simulink model "nonlineardtm"  (R2018b)
settings: configuration reference "Physics" (kept outside this file)
model workspace (MAT data in the model file):
  MCOS : class17 (value not decoded)
undefined symbols (not defined in the file): Aerodynamics, Aligning, Antisway, Brakes, Compliance, ContactPatch, Environment, k1_TireFB_PT1, k1_WheelsFB_PT1, k2_TireFB_PT1, Kinematics, Lateral, Longitudinal, normalizeAngle, omega0_K_Vehicle_radps, omega0_Wheels_radps, Overturning, p_Tires_Pa, Rolling, Scaling, SensorData, Structural, TireSimulation, Turnslip, v0_K_Vehicle_mps, v0z_Wheels_mps, VehicleData, Vertical, Wheels, x0_verticaldynamics, z0_TireDeflection_m
libraries: vehdynlibtire x4, vehdynlibsuspension x2, vrlib x1, vehdynlibeom x1
(part 5 of 5)

== system nonlineardtm/Nonlinear Dual Track Model/Subsystem11/Subsystem10 ==
  Alpha : Inport
  Reshape2 : Reshape  OutputDimensionality=Row vector (2-D)
  Selector : Selector  NumberOfDimensions=2  InputPortWidth=12  IndexOptions=Index vector (dialog),Index vector (dialog)  Indices=[1],1  OutputSizes=1,1
  Selector1 : Selector  NumberOfDimensions=2  InputPortWidth=12  IndexOptions=Index vector (dialog),Index vector (dialog)  Indices=1,2  OutputSizes=1,1
  Selector2 : Selector  NumberOfDimensions=2  InputPortWidth=12  IndexOptions=Index vector (dialog),Index vector (dialog)  Indices=1,3  OutputSizes=1,1
  Selector3 : Selector  NumberOfDimensions=2  InputPortWidth=12  IndexOptions=Index vector (dialog),Index vector (dialog)  Indices=1,3  OutputSizes=1,1
  Transfer Fcn1 : TransferFcn  Denominator=[k1_TireFB_PT1(2) 1]
  Transfer Fcn10 : TransferFcn  Denominator=[k1_TireFB_PT1(1) 1]
  Transfer Fcn11 : TransferFcn  Denominator=[k1_TireFB_PT1(1) 1]
  Transfer Fcn9 : TransferFcn  Denominator=[k1_TireFB_PT1(2) 1]
  Vector Concatenate : Concatenate  NumInputs=4
  alpha_ji_rad : Outport
  wires:
  Transfer Fcn1/1 -> Vector Concatenate/4
  Selector3/1 -> Transfer Fcn1/1
  Transfer Fcn9/1 -> Vector Concatenate/3
  Reshape2/1 -> alpha_ji_rad/1
  Alpha/1 -> Selector/1, Selector1/1, Selector2/1, Selector3/1
  Selector/1 -> Transfer Fcn11/1
  Selector2/1 -> Transfer Fcn9/1
  Selector1/1 -> Transfer Fcn10/1
  Transfer Fcn11/1 -> Vector Concatenate/1
  Transfer Fcn10/1 -> Vector Concatenate/2
  Vector Concatenate/1 -> Reshape2/1

== system nonlineardtm/Nonlinear Dual Track Model/Subsystem11/Subsystem14 ==
  z : Inport
  Reshape2 : Reshape  OutputDimensionality=Row vector (2-D)
  Selector : Selector  NumberOfDimensions=2  InputPortWidth=12  IndexOptions=Index vector (dialog),Index vector (dialog)  Indices=[1],1  OutputSizes=1,1
  Selector1 : Selector  NumberOfDimensions=2  InputPortWidth=12  IndexOptions=Index vector (dialog),Index vector (dialog)  Indices=1,2  OutputSizes=1,1
  Selector2 : Selector  NumberOfDimensions=2  InputPortWidth=12  IndexOptions=Index vector (dialog),Index vector (dialog)  Indices=1,3  OutputSizes=1,1
  Selector3 : Selector  NumberOfDimensions=2  InputPortWidth=12  IndexOptions=Index vector (dialog),Index vector (dialog)  Indices=1,3  OutputSizes=1,1
  Transfer Fcn1 : TransferFcn  Denominator=[k2_TireFB_PT1(2) 1]
  Transfer Fcn10 : TransferFcn  Denominator=[k2_TireFB_PT1(1) 1]
  Transfer Fcn11 : TransferFcn  Denominator=[k2_TireFB_PT1(1) 1]
  Transfer Fcn9 : TransferFcn  Denominator=[k2_TireFB_PT1(2) 1]
  Vector Concatenate : Concatenate  NumInputs=4
  rz_Tji_Rji_m : Outport
  wires:
  Vector Concatenate/1 -> Reshape2/1
  Transfer Fcn10/1 -> Vector Concatenate/2
  Transfer Fcn11/1 -> Vector Concatenate/1
  Selector1/1 -> Transfer Fcn10/1
  Selector2/1 -> Transfer Fcn9/1
  Selector/1 -> Transfer Fcn11/1
  z/1 -> Selector3/1, Selector2/1, Selector1/1, Selector/1
  Reshape2/1 -> rz_Tji_Rji_m/1
  Transfer Fcn9/1 -> Vector Concatenate/3
  Selector3/1 -> Transfer Fcn1/1
  Transfer Fcn1/1 -> Vector Concatenate/4

== system nonlineardtm/Nonlinear Dual Track Model/Subsystem11/Subsystem2 ==
  zdot : Inport
  Reshape2 : Reshape  OutputDimensionality=Row vector (2-D)
  Selector : Selector  NumberOfDimensions=2  InputPortWidth=12  IndexOptions=Index vector (dialog),Index vector (dialog)  Indices=[1],1  OutputSizes=1,1
  Selector1 : Selector  NumberOfDimensions=2  InputPortWidth=12  IndexOptions=Index vector (dialog),Index vector (dialog)  Indices=1,2  OutputSizes=1,1
  Selector2 : Selector  NumberOfDimensions=2  InputPortWidth=12  IndexOptions=Index vector (dialog),Index vector (dialog)  Indices=1,3  OutputSizes=1,1
  Selector3 : Selector  NumberOfDimensions=2  InputPortWidth=12  IndexOptions=Index vector (dialog),Index vector (dialog)  Indices=1,3  OutputSizes=1,1
  Transfer Fcn1 : TransferFcn  Denominator=[k2_TireFB_PT1(2) 1]
  Transfer Fcn10 : TransferFcn  Denominator=[k2_TireFB_PT1(1) 1]
  Transfer Fcn11 : TransferFcn  Denominator=[k2_TireFB_PT1(1) 1]
  Transfer Fcn9 : TransferFcn  Denominator=[k2_TireFB_PT1(2) 1]
  Vector Concatenate : Concatenate  NumInputs=4
  vz_Tji_Rji_mps : Outport
  wires:
  Transfer Fcn1/1 -> Vector Concatenate/4
  Selector3/1 -> Transfer Fcn1/1
  Transfer Fcn9/1 -> Vector Concatenate/3
  Reshape2/1 -> vz_Tji_Rji_mps/1
  zdot/1 -> Selector/1, Selector1/1, Selector2/1, Selector3/1
  Selector/1 -> Transfer Fcn11/1
  Selector2/1 -> Transfer Fcn9/1
  Selector1/1 -> Transfer Fcn10/1
  Transfer Fcn11/1 -> Vector Concatenate/1
  Transfer Fcn10/1 -> Vector Concatenate/2
  Vector Concatenate/1 -> Reshape2/1

== system nonlineardtm/Nonlinear Dual Track Model/Subsystem11/Subsystem3 ==
  Re : Inport
  Reshape2 : Reshape  OutputDimensionality=Row vector (2-D)
  Selector : Selector  NumberOfDimensions=2  InputPortWidth=12  IndexOptions=Index vector (dialog),Index vector (dialog)  Indices=[1],1  OutputSizes=1,1
  Selector1 : Selector  NumberOfDimensions=2  InputPortWidth=12  IndexOptions=Index vector (dialog),Index vector (dialog)  Indices=1,2  OutputSizes=1,1
  Selector2 : Selector  NumberOfDimensions=2  InputPortWidth=12  IndexOptions=Index vector (dialog),Index vector (dialog)  Indices=1,3  OutputSizes=1,1
  Selector3 : Selector  NumberOfDimensions=2  InputPortWidth=12  IndexOptions=Index vector (dialog),Index vector (dialog)  Indices=1,3  OutputSizes=1,1
  Transfer Fcn1 : TransferFcn  Denominator=[k2_TireFB_PT1(2) 1]
  Transfer Fcn10 : TransferFcn  Denominator=[k2_TireFB_PT1(1) 1]
  Transfer Fcn11 : TransferFcn  Denominator=[k2_TireFB_PT1(1) 1]
  Transfer Fcn9 : TransferFcn  Denominator=[k2_TireFB_PT1(2) 1]
  Vector Concatenate : Concatenate  NumInputs=4
  re_ji_m : Outport
  wires:
  Vector Concatenate/1 -> Reshape2/1
  Transfer Fcn10/1 -> Vector Concatenate/2
  Transfer Fcn11/1 -> Vector Concatenate/1
  Selector1/1 -> Transfer Fcn10/1
  Selector2/1 -> Transfer Fcn9/1
  Selector/1 -> Transfer Fcn11/1
  Re/1 -> Selector3/1, Selector2/1, Selector1/1, Selector/1
  Reshape2/1 -> re_ji_m/1
  Transfer Fcn9/1 -> Vector Concatenate/3
  Selector3/1 -> Transfer Fcn1/1
  Transfer Fcn1/1 -> Vector Concatenate/4

== system nonlineardtm/Nonlinear Dual Track Model/Subsystem11/Subsystem6 ==
  F : Inport
  Matrix Concatenate : Concatenate  NumInputs=3  Mode=Multidimensional array
  Reshape2 : Reshape  OutputDimensionality=Row vector (2-D)
  Reshape3 : Reshape  OutputDimensionality=Row vector (2-D)
  Reshape4 : Reshape  OutputDimensionality=Row vector (2-D)
  Selector : Selector  NumberOfDimensions=2  InputPortWidth=12  IndexOptions=Index vector (dialog),Index vector (dialog)  Indices=[1],1  OutputSizes=1,1
  Selector1 : Selector  NumberOfDimensions=2  InputPortWidth=12  IndexOptions=Index vector (dialog),Index vector (dialog)  Indices=1,2  OutputSizes=1,1
  Selector12 : Selector  NumberOfDimensions=2  InputPortWidth=12  IndexOptions=Index vector (dialog),Index vector (dialog)  Indices=2,1  OutputSizes=1,1
  Selector13 : Selector  NumberOfDimensions=2  InputPortWidth=12  IndexOptions=Index vector (dialog),Index vector (dialog)  Indices=2,2  OutputSizes=1,1
  Selector14 : Selector  NumberOfDimensions=2  InputPortWidth=12  IndexOptions=Index vector (dialog),Index vector (dialog)  Indices=2,3  OutputSizes=1,1
  Selector15 : Selector  NumberOfDimensions=2  InputPortWidth=12  IndexOptions=Index vector (dialog),Index vector (dialog)  Indices=2,4  OutputSizes=1,1
  Selector16 : Selector  NumberOfDimensions=2  InputPortWidth=12  IndexOptions=Index vector (dialog),Index vector (dialog)  Indices=3,1  OutputSizes=1,1
  Selector17 : Selector  NumberOfDimensions=2  InputPortWidth=12  IndexOptions=Index vector (dialog),Index vector (dialog)  Indices=3,2  OutputSizes=1,1
  Selector18 : Selector  NumberOfDimensions=2  InputPortWidth=12  IndexOptions=Index vector (dialog),Index vector (dialog)  Indices=3,3  OutputSizes=1,1
  Selector19 : Selector  NumberOfDimensions=2  InputPortWidth=12  IndexOptions=Index vector (dialog),Index vector (dialog)  Indices=3,4  OutputSizes=1,1
  Selector2 : Selector  NumberOfDimensions=2  InputPortWidth=12  IndexOptions=Index vector (dialog),Index vector (dialog)  Indices=1,3  OutputSizes=1,1
  Selector3 : Selector  NumberOfDimensions=2  InputPortWidth=12  IndexOptions=Index vector (dialog),Index vector (dialog)  Indices=1,4  OutputSizes=1,1
  Transfer Fcn{1,4..5,8..9,11} (6 alike) : TransferFcn  Denominator=[k1_TireFB_PT1(1) 1]
  Transfer Fcn{2..3,6..7,10,12} (6 alike) : TransferFcn  Denominator=[k1_TireFB_PT1(2) 1]
  Vector Concatenate : Concatenate  NumInputs=4
  Vector Concatenate1 : Concatenate  NumInputs=4
  Vector Concatenate2 : Concatenate  NumInputs=4
  F_Tji_Tji_N : Outport
  wires:
  Reshape4/1 -> Matrix Concatenate/3
  Reshape3/1 -> Matrix Concatenate/2
  Reshape2/1 -> Matrix Concatenate/1
  Vector Concatenate2/1 -> Reshape4/1
  Vector Concatenate1/1 -> Reshape3/1
  Vector Concatenate/1 -> Reshape2/1
  Transfer Fcn6/1 -> Vector Concatenate1/3
  Transfer Fcn7/1 -> Vector Concatenate1/4
  Transfer Fcn8/1 -> Vector Concatenate2/1
  Transfer Fcn9/1 -> Vector Concatenate2/2
  Transfer Fcn12/1 -> Vector Concatenate2/4
  Transfer Fcn10/1 -> Vector Concatenate2/3
  Transfer Fcn5/1 -> Vector Concatenate1/2
  Transfer Fcn4/1 -> Vector Concatenate1/1
  Transfer Fcn3/1 -> Vector Concatenate/4
  Transfer Fcn2/1 -> Vector Concatenate/3
  Transfer Fcn1/1 -> Vector Concatenate/2
  Transfer Fcn11/1 -> Vector Concatenate/1
  Selector19/1 -> Transfer Fcn12/1
  Selector18/1 -> Transfer Fcn10/1
  Selector17/1 -> Transfer Fcn9/1
  Selector16/1 -> Transfer Fcn8/1
  Selector12/1 -> Transfer Fcn4/1
  Selector13/1 -> Transfer Fcn5/1
  Selector14/1 -> Transfer Fcn6/1
  Selector15/1 -> Transfer Fcn7/1
  Selector3/1 -> Transfer Fcn3/1
  Selector1/1 -> Transfer Fcn1/1
  Selector2/1 -> Transfer Fcn2/1
  Selector/1 -> Transfer Fcn11/1
  F/1 -> Selector1/1, Selector2/1, Selector3/1, Selector19/1, Selector18/1, Selector17/1, Selector16/1, Selector15/1, Selector14/1, Selector13/1, Selector12/1, Selector/1
  Matrix Concatenate/1 -> F_Tji_Tji_N/1

== system nonlineardtm/Nonlinear Dual Track Model/Subsystem11/Subsystem8 ==
  omega : Inport
  Reshape2 : Reshape  OutputDimensionality=Row vector (2-D)
  Selector : Selector  NumberOfDimensions=2  InputPortWidth=12  IndexOptions=Index vector (dialog),Index vector (dialog)  Indices=[1],1  OutputSizes=1,1
  Selector1 : Selector  NumberOfDimensions=2  InputPortWidth=12  IndexOptions=Index vector (dialog),Index vector (dialog)  Indices=1,2  OutputSizes=1,1
  Selector2 : Selector  NumberOfDimensions=2  InputPortWidth=12  IndexOptions=Index vector (dialog),Index vector (dialog)  Indices=1,3  OutputSizes=1,1
  Selector3 : Selector  NumberOfDimensions=2  InputPortWidth=12  IndexOptions=Index vector (dialog),Index vector (dialog)  Indices=1,4  OutputSizes=1,1
  Transfer Fcn1 : TransferFcn  Denominator=[k1_WheelsFB_PT1(2) 1]
  Transfer Fcn10 : TransferFcn  Denominator=[k1_WheelsFB_PT1(1) 1]
  Transfer Fcn11 : TransferFcn  Denominator=[k1_WheelsFB_PT1(1) 1]
  Transfer Fcn9 : TransferFcn  Denominator=[k1_WheelsFB_PT1(2) 1]
  Vector Concatenate : Concatenate  NumInputs=4
  omegay_Rji_Rji_radps : Outport
  wires:
  Transfer Fcn1/1 -> Vector Concatenate/4
  Selector3/1 -> Transfer Fcn1/1
  Transfer Fcn9/1 -> Vector Concatenate/3
  Reshape2/1 -> omegay_Rji_Rji_radps/1
  omega/1 -> Selector/1, Selector1/1, Selector2/1, Selector3/1
  Selector/1 -> Transfer Fcn11/1
  Selector2/1 -> Transfer Fcn9/1
  Selector1/1 -> Transfer Fcn10/1
  Transfer Fcn11/1 -> Vector Concatenate/1
  Transfer Fcn10/1 -> Vector Concatenate/2
  Vector Concatenate/1 -> Reshape2/1

== system nonlineardtm/Nonlinear Dual Track Model/Subsystem11/Subsystem9 ==
  Kappa : Inport
  Reshape2 : Reshape  OutputDimensionality=Row vector (2-D)
  Selector : Selector  NumberOfDimensions=2  InputPortWidth=12  IndexOptions=Index vector (dialog),Index vector (dialog)  Indices=[1],1  OutputSizes=1,1
  Selector1 : Selector  NumberOfDimensions=2  InputPortWidth=12  IndexOptions=Index vector (dialog),Index vector (dialog)  Indices=1,2  OutputSizes=1,1
  Selector2 : Selector  NumberOfDimensions=2  InputPortWidth=12  IndexOptions=Index vector (dialog),Index vector (dialog)  Indices=1,3  OutputSizes=1,1
  Selector3 : Selector  NumberOfDimensions=2  InputPortWidth=12  IndexOptions=Index vector (dialog),Index vector (dialog)  Indices=1,3  OutputSizes=1,1
  Transfer Fcn1 : TransferFcn  Denominator=[k1_TireFB_PT1(2) 1]
  Transfer Fcn10 : TransferFcn  Denominator=[k1_TireFB_PT1(1) 1]
  Transfer Fcn11 : TransferFcn  Denominator=[k1_TireFB_PT1(1) 1]
  Transfer Fcn9 : TransferFcn  Denominator=[k1_TireFB_PT1(2) 1]
  Vector Concatenate : Concatenate  NumInputs=4
  kappa_ji : Outport
  wires:
  Vector Concatenate/1 -> Reshape2/1
  Transfer Fcn10/1 -> Vector Concatenate/2
  Transfer Fcn11/1 -> Vector Concatenate/1
  Selector1/1 -> Transfer Fcn10/1
  Selector2/1 -> Transfer Fcn9/1
  Selector/1 -> Transfer Fcn11/1
  Kappa/1 -> Selector3/1, Selector2/1, Selector1/1, Selector/1
  Reshape2/1 -> kappa_ji/1
  Transfer Fcn9/1 -> Vector Concatenate/3
  Selector3/1 -> Transfer Fcn1/1
  Transfer Fcn1/1 -> Vector Concatenate/4

== system nonlineardtm/Nonlinear Dual Track Model/Suspension System/Rearrange Signals ==
  Info f : Inport
  Info r : Inport  Port=2
  Bus Selector1 : BusSelector  OutputSignals=VehF
  Bus Selector10 : BusSelector  OutputSignals=WhlF
  Bus Selector13 : BusSelector  OutputSignals=WhlV
  Bus Selector16 : BusSelector  OutputSignals=WhlV
  Bus Selector17 : BusSelector  OutputSignals=WhlAng
  Bus Selector2 : BusSelector  OutputSignals=VehF
  Bus Selector20 : BusSelector  OutputSignals=WhlAng
  Bus Selector21 : BusSelector  OutputSignals=Height
  Bus Selector24 : BusSelector  OutputSignals=Height
  Bus Selector5 : BusSelector  OutputSignals=VehM
  Bus Selector6 : BusSelector  OutputSignals=VehM
  Bus Selector9 : BusSelector  OutputSignals=WhlF
  Matrix Concatenate{,1..5} (6 alike) : Concatenate  Mode=Multidimensional array  ConcatenateDimension=2
  VehF : Outport
  VehM : Outport  Port=2
  WhlF : Outport  Port=3
  WhlV : Outport  Port=4
  WhlAng : Outport  Port=5
  SuspH : Outport  Port=6
  wires:
  Bus Selector2/1 -> Matrix Concatenate/1  "<VehF>"
  Bus Selector1/1 -> Matrix Concatenate/2  "<VehF>"
  Bus Selector5/1 -> Matrix Concatenate1/2  "<VehM>"
  Bus Selector6/1 -> Matrix Concatenate1/1  "<VehM>"
  Bus Selector10/1 -> Matrix Concatenate2/1  "<WhlF>"
  Bus Selector9/1 -> Matrix Concatenate2/2  "<WhlF>"
  Bus Selector16/1 -> Matrix Concatenate3/2  "<WhlV>"
  Bus Selector13/1 -> Matrix Concatenate3/1  "<WhlV>"
  Bus Selector17/1 -> Matrix Concatenate4/1  "<WhlAng>"
  Bus Selector20/1 -> Matrix Concatenate4/2  "<WhlAng>"
  Bus Selector24/1 -> Matrix Concatenate5/2  "<Height>"
  Bus Selector21/1 -> Matrix Concatenate5/1  "<Height>"
  Info r/1 -> Bus Selector24/1, Bus Selector20/1, Bus Selector16/1, Bus Selector9/1, Bus Selector5/1, Bus Selector1/1
  Info f/1 -> Bus Selector2/1, Bus Selector21/1, Bus Selector17/1, Bus Selector13/1, Bus Selector10/1, Bus Selector6/1
  Matrix Concatenate/1 -> VehF/1
  Matrix Concatenate1/1 -> VehM/1
  Matrix Concatenate2/1 -> WhlF/1
  Matrix Concatenate3/1 -> WhlV/1
  Matrix Concatenate4/1 -> WhlAng/1
  Matrix Concatenate5/1 -> SuspH/1

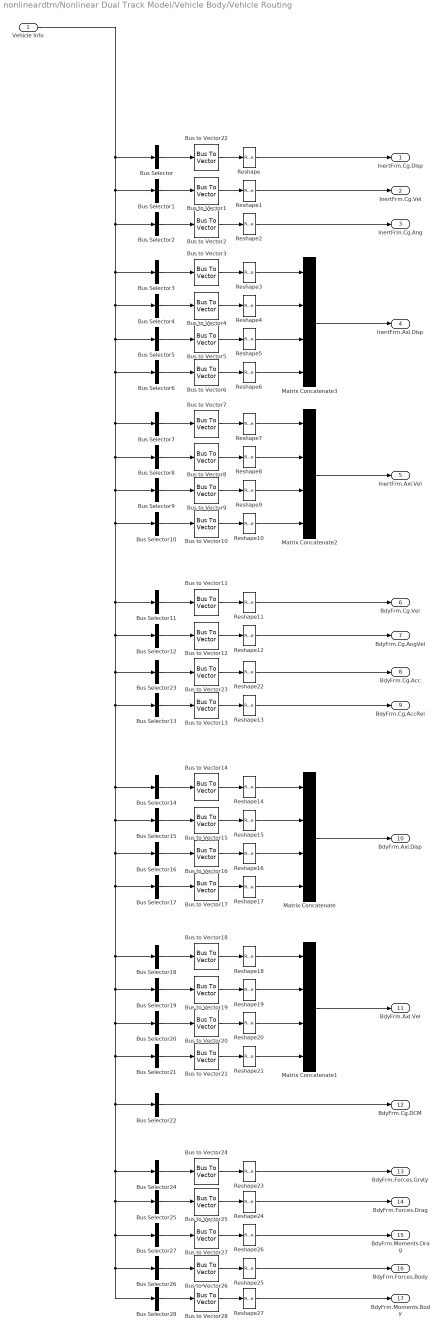
== system nonlineardtm/Nonlinear Dual Track Model/Vehicle Body/Vehicle Routing ==
  Vehicle Info : Inport
  Bus Selector : BusSelector  OutputSignals=InertFrm.Cg.Disp.X,InertFrm.Cg.Disp.Y,InertFrm.Cg.Disp.Z  OutputAsBus=on
  Bus Selector1 : BusSelector  OutputSignals=InertFrm.Cg.Vel.Xdot,InertFrm.Cg.Vel.Ydot,InertFrm.Cg.Vel.Zdot  OutputAsBus=on
  Bus Selector10 : BusSelector  OutputSignals=InertFrm.RearAxl.Rght.Vel.Xdot,InertFrm.RearAxl.Rght.Vel.Ydot,InertFrm.RearAxl.Rght.Vel.Zdot  OutputAsBus=on
  Bus Selector11 : BusSelector  OutputSignals=BdyFrm.Cg.Vel.xdot,BdyFrm.Cg.Vel.ydot,BdyFrm.Cg.Vel.zdot  OutputAsBus=on
  Bus Selector12 : BusSelector  OutputSignals=BdyFrm.Cg.AngVel.p,BdyFrm.Cg.AngVel.q,BdyFrm.Cg.AngVel.r  OutputAsBus=on
  Bus Selector13 : BusSelector  OutputSignals=BdyFrm.Cg.Acc.xddot,BdyFrm.Cg.Acc.yddot,BdyFrm.Cg.Acc.zddot  OutputAsBus=on
  Bus Selector14 : BusSelector  OutputSignals=BdyFrm.FrntAxl.Lft.Disp.x,BdyFrm.FrntAxl.Lft.Disp.y,BdyFrm.FrntAxl.Lft.Disp.z  OutputAsBus=on
  Bus Selector15 : BusSelector  OutputSignals=BdyFrm.FrntAxl.Rght.Disp.x,BdyFrm.FrntAxl.Rght.Disp.y,BdyFrm.FrntAxl.Rght.Disp.z  OutputAsBus=on
  Bus Selector16 : BusSelector  OutputSignals=BdyFrm.RearAxl.Lft.Disp.x,BdyFrm.RearAxl.Lft.Disp.y,BdyFrm.RearAxl.Lft.Disp.z  OutputAsBus=on
  Bus Selector17 : BusSelector  OutputSignals=BdyFrm.RearAxl.Rght.Disp.x,BdyFrm.RearAxl.Rght.Disp.y,BdyFrm.RearAxl.Rght.Disp.z  OutputAsBus=on
  Bus Selector18 : BusSelector  OutputSignals=BdyFrm.FrntAxl.Lft.Vel.xdot,BdyFrm.FrntAxl.Lft.Vel.ydot,BdyFrm.FrntAxl.Lft.Vel.zdot  OutputAsBus=on
  Bus Selector19 : BusSelector  OutputSignals=BdyFrm.FrntAxl.Rght.Vel.xdot,BdyFrm.FrntAxl.Rght.Vel.ydot,BdyFrm.FrntAxl.Rght.Vel.zdot  OutputAsBus=on
  Bus Selector2 : BusSelector  OutputSignals=InertFrm.Cg.Ang.phi,InertFrm.Cg.Ang.theta,InertFrm.Cg.Ang.psi  OutputAsBus=on
  Bus Selector20 : BusSelector  OutputSignals=BdyFrm.RearAxl.Lft.Vel.xdot,BdyFrm.RearAxl.Lft.Vel.ydot,BdyFrm.RearAxl.Lft.Vel.zdot  OutputAsBus=on
  Bus Selector21 : BusSelector  OutputSignals=BdyFrm.RearAxl.Rght.Vel.xdot,BdyFrm.RearAxl.Rght.Vel.ydot,BdyFrm.RearAxl.Rght.Vel.zdot  OutputAsBus=on
  Bus Selector22 : BusSelector  OutputSignals=BdyFrm.Cg.DCM  OutputAsBus=on
  Bus Selector23 : BusSelector  OutputSignals=BdyFrm.Cg.Acc.ax,BdyFrm.Cg.Acc.ay,BdyFrm.Cg.Acc.az  OutputAsBus=on
  Bus Selector24 : BusSelector  OutputSignals=BdyFrm.Forces.Grvty.Fx,BdyFrm.Forces.Grvty.Fy,BdyFrm.Forces.Grvty.Fz  OutputAsBus=on
  Bus Selector25 : BusSelector  OutputSignals=BdyFrm.Forces.Drag.Fx,BdyFrm.Forces.Drag.Fy,BdyFrm.Forces.Drag.Fz  OutputAsBus=on
  Bus Selector26 : BusSelector  OutputSignals=BdyFrm.Forces.Body.Fx,BdyFrm.Forces.Body.Fy,BdyFrm.Forces.Body.Fz  OutputAsBus=on
  Bus Selector27 : BusSelector  OutputSignals=BdyFrm.Moments.Drag.Mx,BdyFrm.Moments.Drag.My,BdyFrm.Moments.Drag.Mz  OutputAsBus=on
  Bus Selector28 : BusSelector  OutputSignals=BdyFrm.Moments.Body.Mx,BdyFrm.Moments.Body.My,BdyFrm.Moments.Body.Mz  OutputAsBus=on
  Bus Selector3 : BusSelector  OutputSignals=InertFrm.FrntAxl.Lft.Disp.X,InertFrm.FrntAxl.Lft.Disp.Y,InertFrm.FrntAxl.Lft.Disp.Z  OutputAsBus=on
  Bus Selector4 : BusSelector  OutputSignals=InertFrm.FrntAxl.Rght.Disp.X,InertFrm.FrntAxl.Rght.Disp.Y,InertFrm.FrntAxl.Rght.Disp.Z  OutputAsBus=on
  Bus Selector5 : BusSelector  OutputSignals=InertFrm.RearAxl.Lft.Disp.X,InertFrm.RearAxl.Lft.Disp.Y,InertFrm.RearAxl.Lft.Disp.Z  OutputAsBus=on
  Bus Selector6 : BusSelector  OutputSignals=InertFrm.RearAxl.Rght.Disp.X,InertFrm.RearAxl.Rght.Disp.Y,InertFrm.RearAxl.Rght.Disp.Z  OutputAsBus=on
  Bus Selector7 : BusSelector  OutputSignals=InertFrm.FrntAxl.Lft.Vel.Xdot,InertFrm.FrntAxl.Lft.Vel.Ydot,InertFrm.FrntAxl.Lft.Vel.Zdot  OutputAsBus=on
  Bus Selector8 : BusSelector  OutputSignals=InertFrm.FrntAxl.Rght.Vel.Xdot,InertFrm.FrntAxl.Rght.Vel.Ydot,InertFrm.FrntAxl.Rght.Vel.Zdot  OutputAsBus=on
  Bus Selector9 : BusSelector  OutputSignals=InertFrm.RearAxl.Lft.Vel.Xdot,InertFrm.RearAxl.Lft.Vel.Ydot,InertFrm.RearAxl.Lft.Vel.Zdot  OutputAsBus=on
  Bus to Vector{1..28} (28 alike) : BusToVector
  Matrix Concatenate{,1..3} (4 alike) : Concatenate  NumInputs=4  Mode=Multidimensional array  ConcatenateDimension=2
  Reshape{,1..27} (28 alike) : Reshape  OutputDimensionality=Column vector (2-D)
  InertFrm.Cg.Disp : Outport
  InertFrm.Cg.Vel : Outport  Port=2
  InertFrm.Cg.Ang : Outport  Port=3
  InertFrm.Axl.Disp : Outport  Port=4
  InertFrm.Axl.Vel : Outport  Port=5
  BdyFrm.Cg.Vel : Outport  Port=6
  BdyFrm.Cg.AngVel : Outport  Port=7
  BdyFrm.Cg.Acc : Outport  Port=8
  BdyFrm.Cg.AccRel : Outport  Port=9
  BdyFrm.Axl.Disp : Outport  Port=10
  BdyFrm.Axl.Vel : Outport  Port=11
  BdyFrm.Cg.DCM : Outport  Port=12
  BdyFrm.Forces.Grvty : Outport  Port=13
  BdyFrm.Forces.Drag : Outport  Port=14
  BdyFrm.Moments.Drag : Outport  Port=15
  BdyFrm.Forces.Body : Outport  Port=16
  BdyFrm.Moments.Body : Outport  Port=17
  wires:
  Bus to Vector22/1 -> Reshape/1
  Bus to Vector1/1 -> Reshape1/1
  Bus Selector1/1 -> Bus to Vector1/1
  Bus Selector2/1 -> Bus to Vector2/1
  Bus to Vector2/1 -> Reshape2/1
  Bus to Vector3/1 -> Reshape3/1
  Bus Selector3/1 -> Bus to Vector3/1
  Bus Selector4/1 -> Bus to Vector4/1
  Bus to Vector4/1 -> Reshape4/1
  Bus to Vector5/1 -> Reshape5/1
  Bus Selector5/1 -> Bus to Vector5/1
  Bus Selector6/1 -> Bus to Vector6/1
  Bus to Vector6/1 -> Reshape6/1
  Bus to Vector7/1 -> Reshape7/1
  Bus Selector7/1 -> Bus to Vector7/1
  Bus Selector8/1 -> Bus to Vector8/1
  Bus to Vector8/1 -> Reshape8/1
  Bus to Vector9/1 -> Reshape9/1
  Bus Selector9/1 -> Bus to Vector9/1
  Bus Selector10/1 -> Bus to Vector10/1
  Bus to Vector10/1 -> Reshape10/1
  Bus Selector13/1 -> Bus to Vector13/1
  Bus to Vector13/1 -> Reshape13/1
  Bus to Vector12/1 -> Reshape12/1
  Bus Selector12/1 -> Bus to Vector12/1
  Bus Selector11/1 -> Bus to Vector11/1
  Bus to Vector11/1 -> Reshape11/1
  Bus to Vector14/1 -> Reshape14/1
  Bus Selector14/1 -> Bus to Vector14/1
  Bus Selector15/1 -> Bus to Vector15/1
  Bus to Vector15/1 -> Reshape15/1
  Bus to Vector16/1 -> Reshape16/1
  Bus Selector16/1 -> Bus to Vector16/1
  Bus Selector17/1 -> Bus to Vector17/1
  Bus to Vector17/1 -> Reshape17/1
  Bus to Vector21/1 -> Reshape21/1
  Bus Selector21/1 -> Bus to Vector21/1
  Bus Selector20/1 -> Bus to Vector20/1
  Bus to Vector20/1 -> Reshape20/1
  Bus to Vector19/1 -> Reshape19/1
  Bus Selector19/1 -> Bus to Vector19/1
  Bus Selector18/1 -> Bus to Vector18/1
  Bus to Vector18/1 -> Reshape18/1
  Bus Selector/1 -> Bus to Vector22/1
  Reshape3/1 -> Matrix Concatenate3/1
  Reshape4/1 -> Matrix Concatenate3/2
  Reshape5/1 -> Matrix Concatenate3/3
  Reshape6/1 -> Matrix Concatenate3/4
  Reshape7/1 -> Matrix Concatenate2/1
  Reshape8/1 -> Matrix Concatenate2/2
  Reshape9/1 -> Matrix Concatenate2/3
  Reshape10/1 -> Matrix Concatenate2/4
  Reshape14/1 -> Matrix Concatenate/1
  Reshape15/1 -> Matrix Concatenate/2
  Reshape16/1 -> Matrix Concatenate/3
  Reshape17/1 -> Matrix Concatenate/4
  Reshape18/1 -> Matrix Concatenate1/1
  Reshape19/1 -> Matrix Concatenate1/2
  Reshape20/1 -> Matrix Concatenate1/3
  Reshape21/1 -> Matrix Concatenate1/4
  Bus to Vector23/1 -> Reshape22/1
  Bus Selector23/1 -> Bus to Vector23/1
  Bus Selector24/1 -> Bus to Vector24/1
  Bus to Vector24/1 -> Reshape23/1
  Bus to Vector25/1 -> Reshape24/1
  Bus Selector25/1 -> Bus to Vector25/1
  Bus Selector26/1 -> Bus to Vector26/1
  Bus to Vector26/1 -> Reshape25/1
  Bus to Vector27/1 -> Reshape26/1
  Bus Selector27/1 -> Bus to Vector27/1
  Bus Selector28/1 -> Bus to Vector28/1
  Bus to Vector28/1 -> Reshape27/1
  Vehicle Info/1 -> Bus Selector14/1, Bus Selector15/1, Bus Selector16/1, Bus Selector17/1, Bus Selector18/1, Bus Selector19/1, Bus Selector28/1, Bus Selector26/1, Bus Selector27/1, Bus Selector25/1, Bus Selector24/1, Bus Selector22/1, Bus Selector21/1, Bus Selector20/1, Bus Selector13/1, Bus Selector23/1, Bus Selector12/1, Bus Selector11/1, Bus Selector10/1, Bus Selector9/1, Bus Selector8/1, Bus Selector7/1, Bus Selector6/1, Bus Selector5/1, Bus Selector4/1, Bus Selector3/1, Bus Selector2/1, Bus Selector1/1, Bus Selector/1
  Reshape/1 -> InertFrm.Cg.Disp/1
  Reshape1/1 -> InertFrm.Cg.Vel/1
  Reshape2/1 -> InertFrm.Cg.Ang/1
  Matrix Concatenate3/1 -> InertFrm.Axl.Disp/1
  Matrix Concatenate2/1 -> InertFrm.Axl.Vel/1
  Reshape11/1 -> BdyFrm.Cg.Vel/1
  Reshape12/1 -> BdyFrm.Cg.AngVel/1
  Reshape22/1 -> BdyFrm.Cg.Acc/1
  Reshape13/1 -> BdyFrm.Cg.AccRel/1
  Matrix Concatenate/1 -> BdyFrm.Axl.Disp/1
  Matrix Concatenate1/1 -> BdyFrm.Axl.Vel/1
  Bus Selector22/1 -> BdyFrm.Cg.DCM/1
  Reshape23/1 -> BdyFrm.Forces.Grvty/1
  Reshape24/1 -> BdyFrm.Forces.Drag/1
  Reshape26/1 -> BdyFrm.Moments.Drag/1
  Reshape25/1 -> BdyFrm.Forces.Body/1
  Reshape27/1 -> BdyFrm.Moments.Body/1

== matlab function nonlineardtm/Nonlinear Dual Track Model/Computation Sensor Position and Orientation ==
  data: r_I_IK_m input; r_I_IS1_m output; A_K_I input; r_I_IS2_m output; r_I_IS3_m output; A_S1_I output; A_S2_I output; A_S3_I output; r_K_KS1_m input; r_K_KS2_m input; r_K_KS3_m input; phi0_K_KS1_rad input; phi0_K_KS2_rad input; phi0_K_KS3_rad input
function [r_I_IS1_m,r_I_IS2_m,r_I_IS3_m,A_S1_I,A_S2_I,A_S3_I] = fcn(r_I_IK_m,A_K_I,r_K_KS1_m,r_K_KS2_m,r_K_KS3_m,phi0_K_KS1_rad,phi0_K_KS2_rad,phi0_K_KS3_rad)

[r_I_IS1_m,r_I_IS2_m,r_I_IS3_m,A_S1_I,A_S2_I,A_S3_I] = Transformation_Sensor(r_I_IK_m,A_K_I,r_K_KS1_m,r_K_KS2_m,r_K_KS3_m,phi0_K_KS1_rad,phi0_K_KS2_rad,phi0_K_KS3_rad);

end

== matlab function nonlineardtm/Nonlinear Dual Track Model/Rotation Hardpoint Position from InertialFixed ==
  data: r_I_IAji_m input; r_F_IAji_m output; A_K_I input; A_F_I input
function r_F_IAji_m = fcn(r_I_IAji_m,A_K_I,A_F_I)

r_F_IAji_m = Rotation_Position_FromInertialFixed(r_I_IAji_m,A_K_I,A_F_I);

end

== matlab function nonlineardtm/Nonlinear Dual Track Model/Computation Road Inclination Angles Arkustangens ==
  data: z_I_Ground_m input; rx_I_IAji_m input; ry_I_IAji_m input; chi output; phiz_IK_rad input
function chi = fcn(z_I_Ground_m,rx_I_IAji_m,ry_I_IAji_m,phiz_IK_rad)

[chi] = RoadInclination_Arkustangens(z_I_Ground_m,rx_I_IAji_m,ry_I_IAji_m,phiz_IK_rad);

end

== matlab function nonlineardtm/Nonlinear Dual Track Model/Rotation Hardpoint Velocities from VehicleFixed ==
  data: v_K_IAji_mps input; v_F_IAji_mps output; A_K_F input
function v_F_IAji_mps = fcn(v_K_IAji_mps,A_K_F)

[v_F_IAji_mps] = Rotation_Velocity_FromVehicleFixed(v_K_IAji_mps,A_K_F);

end

== matlab function nonlineardtm/Nonlinear Dual Track Model/Rotation Angular Velocities VehicleFixed to TireFixed ==
  data: omega_K_IK_radps input; A_K_F input; omega_Tji_ITji_radps output; A_down_up input
function omega_Tji_ITji_radps = fcn(omega_K_IK_radps,A_K_F,A_down_up)

[omega_Tji_ITji_radps] = Rotation_AngVelocity_ToTireFixed(omega_K_IK_radps,A_K_F,A_down_up);

end

== matlab function nonlineardtm/Nonlinear Dual Track Model/Computation Transformation Matrices ==
  data: phi input; chi input; delta input; A_K_I output; A_K_F output; A_F_I output; A_Rfl_F output; A_Rfr_F output; A_down_up output
function [A_K_I,A_K_F,A_F_I,A_Rfl_F,A_Rfr_F,A_down_up] = fcn(phi,chi,delta)

[A_K_I,A_K_F,A_F_I,A_Rfl_F,A_Rfr_F,A_down_up] = Rotation_Matrices(phi,chi,delta);

end

== matlab function nonlineardtm/Nonlinear Dual Track Model/Rotation Hardpoint Moments to VehicleFixed ==
  data: T_F_Aji_Nm input; T_K_Aji_Nm output; A_K_F input
function T_K_Aji_Nm = fcn(T_F_Aji_Nm,A_K_F)

[T_K_Aji_Nm] = Rotation_ForceMoment_ToVehicleFixed(T_F_Aji_Nm,A_K_F);

end

== matlab function nonlineardtm/Nonlinear Dual Track Model/Rotation Hardpoint Forces to VehicleFixed ==
  data: F_F_Aji_N input; F_K_Aji_N output; A_K_F input
function F_K_Aji_N = fcn(F_F_Aji_N,A_K_F)

[F_K_Aji_N] = Rotation_ForceMoment_ToVehicleFixed(F_F_Aji_N,A_K_F);

end

== matlab function nonlineardtm/Nonlinear Dual Track Model/Rotation Road Displacement InertialFrame to TireFixed ==
  data: z_Tji_Ground_m output; r_I_IRji_m output; r_I_ITji_m output; z_I_Ground_m input; A_K_I input; A_F_I input; r_I_IAji_m input; h_ji_m input; re_ji_m input
function [z_Tji_Ground_m,r_I_IRji_m,r_I_ITji_m] = fcn(z_I_Ground_m,A_K_I,A_F_I,r_I_IAji_m,h_ji_m,re_ji_m)

[z_Tji_Ground_m,r_I_IRji_m,r_I_ITji_m] = Rotation_Position_ToTireFixed(z_I_Ground_m,A_K_I,A_F_I,r_I_IAji_m,h_ji_m,re_ji_m);

end

== matlab function nonlineardtm/Nonlinear Dual Track Model/Rotation Forces from TireFixed ==
  data: F_Tji_Tji_N input; F_F_Tji_N output; A_K_F input; A_Rfl_F input; A_Rfr_F input; A_down_up input
function F_F_Tji_N = fcn(F_Tji_Tji_N,A_K_F,A_Rfl_F,A_Rfr_F,A_down_up)

[F_F_Tji_N] = Rotation_ForceMoment_FromTireFixed(F_Tji_Tji_N,A_K_F,A_Rfl_F,A_Rfr_F,A_down_up);

end

== matlab function nonlineardtm/Nonlinear Dual Track Model/Rotation Moments from TireFixed ==
  data: T_Tji_Tji_Nm input; T_F_Tji_Nm output; A_K_F input; A_Rfl_F input; A_Rfr_F input; A_down_up input
function T_F_Tji_Nm = fcn(T_Tji_Tji_Nm,A_K_F,A_Rfl_F,A_Rfr_F,A_down_up)

[T_F_Tji_Nm] = Rotation_ForceMoment_FromTireFixed(T_Tji_Tji_Nm,A_K_F,A_Rfl_F,A_Rfr_F,A_down_up);

end

== matlab function nonlineardtm/Nonlinear Dual Track Model/Aerodynamic Lift ==
  data: v_I_Wind_mps input; F_K_Lift_N output; v_K_IK_mps input; A_K_I input; cl_LongitudinalLift input; A_LongitudinalDrag_m2 input; t_Air_K input; p_Air_Pa input
function F_K_Lift_N = fcn(v_I_Wind_mps,v_K_IK_mps,A_K_I,cl_LongitudinalLift,A_LongitudinalDrag_m2,t_Air_K,p_Air_Pa)

%% Computation of Aerodynamic Lift without bistability (change of signs) around zero pitch angle

%% Environmental Parameters
% Reynolds-Constant
R=287.058;
% Environment Density
rho_Air_kgpm3=p_Air_Pa/(R*t_Air_K);

%% Relative Air-Speed (according to MATLAB-documentation)
% Transformation of Wind-velocity  from inertial reference frame into vehicle body reference frame
v_K_Wind_mps=A_K_I*v_I_Wind_mps;
% Relative Air Speed
w=sqrt( (v_K_IK_mps(1)-v_K_Wind_mps(1)).^2 + (v_K_IK_mps(2)-v_K_Wind_mps(2)).^2 +(v_K_Wind_mps(3)).^2 );

%% Computation of Aerodynamic Lift
F_K_Lift_N = [0;0;rho_Air_kgpm3/2*cl_LongitudinalLift.*A_LongitudinalDrag_m2.*w.^2];

== matlab function nonlineardtm/Nonlinear Dual Track Model/Computation Road Inclination Angles Arkussinus ==
  data: z_I_Ground_m input; l_WheelbaseFB_m input; chi output; w_TrackFB_m input; phiz_IK_rad input
function chi = fcn(z_I_Ground_m,l_WheelbaseFB_m,w_TrackFB_m,phiz_IK_rad)

chi = RoadInclination_Arkussinus(z_I_Ground_m,l_WheelbaseFB_m,w_TrackFB_m,phiz_IK_rad);

end

== matlab function nonlineardtm/Nonlinear Dual Track Model/Wheel Inertia according d'Alembert ==
  data: a_K_IK_mps2 input; A_K_F input; F_K_dAlembert_N output; m_WheelsFB_kg input
function F_K_dAlembert_N = fcn(a_K_IK_mps2,A_K_F,m_WheelsFB_kg)

%% Computation of d'Alembert inertia forces of wheel masses
% In order to use the wheel inertia forces according to d'Alembert, set the
% m_VehicleMass_kg of the Vehicle Body 6DOF block to the sprung mass and
% m_WheelsFB_kg of the CombinedSlipWheels 2DOF to the unsprung mass per wheel.

%% Entire Mass of the four wheels (unsprung mass)
m_unsprung_kg = 2*sum(m_WheelsFB_kg);

%% Computation of inertia forces of d'Alembert

% Quarter Vehicle Model along Rear Axle Fixed z-Axis
a_F_IK_mps2 = transpose(A_K_F)*a_K_IK_mps2;
F_F_dAlembert_N = - m_unsprung_kg.*[a_F_IK_mps2(1);a_F_IK_mps2(2);0];
F_K_dAlembert_N = A_K_F*F_F_dAlembert_N;
% Alternatively simplified for small vehicle roll and pitch angles (A_K_F approximates identity)
% F_K_dAlembert_N = - m_unsprung_kg.*[a_K_IK_mps2(1);a_K_IK_mps2(2);0];

% Quarter Vehicle Model along Vehicle Fixed z-Axis
% F_K_dAlembert_N = - m_unsprung_kg.*[a_K_IK_mps2(1);a_K_IK_mps2(2);0];

== matlab function nonlineardtm/Nonlinear Dual Track Model/Rotation Velocities to TireFixed ==
  data: v_F_IRji_mps input; v_Tji_Rji_mps output; A_K_F input; A_Rfl_F input; A_Rfr_F input; A_down_up input
function v_Tji_Rji_mps = fcn(v_F_IRji_mps,A_K_F,A_Rfl_F,A_Rfr_F,A_down_up)

[v_Tji_Rji_mps] = Rotation_Velocity_ToTireFixed(v_F_IRji_mps,A_K_F,A_Rfl_F,A_Rfr_F,A_down_up);

end
